simulink model "ExampleModel"  (R2020b)
settings: Solver=FixedStepAuto  StartTime=0.0  StopTime=Inf  FixedStep=0.010  RelTol=1e-3
undefined symbols (not defined in the file): DiscIntNeverNeededParam
settings Model: Creator=kaebi  LastModifiedBy=kaebi
settings OptimizationCC: DefaultParameterBehavior=Inlined  LocalBlockOutputs=off
settings DebuggingCC: BusObjectLabelMismatch=error
settings RTWCC: Description=TwinCAT GRT Target  SystemTargetFile=TwinCatGrt.tlc  GenCodeOnly=on  TemplateMakefile=tcgrt_msbuild.tmf  TargetLang=C++
settings STFCustomTargetCC: TargetLangStandard=C++03 (ISO)  ConcurrentExecutionCompliant=off  CombineOutputUpdateFcns=on  CodeInterfacePackaging=Reusable function  GRTInterface=off  GenerateAllocFcn=on  SystemTargetFile=TwinCatGrt.tlc
settings GRTTargetCC: TargetLangStandard=C++03 (ISO)  ParMdlRefBuildCompliant=off  CompOptLevelCompliant=off  ConcurrentExecutionCompliant=off  MatFileLogging=off  CodeInterfacePackaging=Reusable function  GenerateAllocFcn=on  UseToolchainInfoCompliant=off  ExtModeMexFile=TcExtModeClient
settings ConfigComp: PLC_OutputDir=delme  PLC_TargetIDE=twincat3

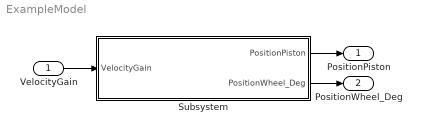
== system ExampleModel ==
  VelocityGain : Inport
  Subsystem : Subsystem  TreatAsAtomicUnit=on
  PositionPiston : Outport
  PositionWheel_Deg : Outport  Port=2
  wires:
  VelocityGain/1 -> Subsystem/1(VelocityGain)
  Subsystem/1(PositionPiston) -> PositionPiston/1
  Subsystem/2(PositionWheel_Deg) -> PositionWheel_Deg/1

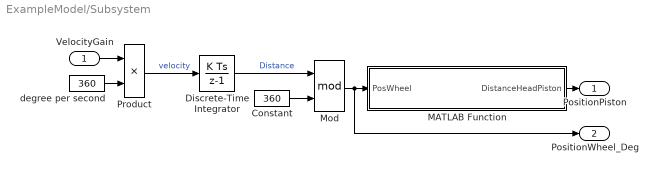
== system ExampleModel/Subsystem ==
  VelocityGain : Inport
  Constant : Constant  Value=360
  Discrete-Time Integrator : DiscreteIntegrator  SampleTime=-1  ICPrevOutput=DiscIntNeverNeededParam  ICPrevScaledInput=DiscIntNeverNeededParam
  MATLAB Function : MATLAB Function  TreatAsAtomicUnit=on
  Mod : Math  Operator=mod  SaturateOnIntegerOverflow=on
  Product : Product
  degree per second : Constant  Value=360
  PositionPiston : Outport
  PositionWheel_Deg : Outport  Port=2
  wires:
  Discrete-Time Integrator/1 -> Mod/1  "Distance"
  Constant/1 -> Mod/2
  Mod/1 -> PositionWheel_Deg/1, MATLAB Function/1(PosWheel)
  degree per second/1 -> Product/2
  VelocityGain/1 -> Product/1
  Product/1 -> Discrete-Time Integrator/1  "velocity"
  MATLAB Function/1(DistanceHeadPiston) -> PositionPiston/1

== matlab function ExampleModel/Subsystem/MATLAB Function ==
  data: PosWheel input; DistanceHeadPiston output
function DistanceHeadPiston = CalcPositionPiston(PosWheel)
    R = 9;
    L = 25;
    K = 13;
    
    DistanceHeadPiston = K + cosd(PosWheel)*R + sqrt(L^2-(sind(PosWheel)*R)^2);


end
